simulink model "proto5"  (R2013b)
settings: Solver=ode45  StartTime=0.0  StopTime=3950  RelTol=1e-3
libraries: xbsIndex_r4 x1250, casper_library_misc x10, xps_library x3
(part 2 of 10)

== system proto5/1st_time ==
  out_reg : Inport
  assert_reg : xbsIndex_r4/Assert  assert_type=on  type_source=Explicitly  gui_display_data_type=Fixed-point  arith_type=Unsigned  n_bits=32  bin_pt=0  preci_type=Single  exp_width=8  frac_width=24  assert_rate=off  rate_source=Explicitly  period=1  output_port=on  block_type=assert
  cast_gw : xbsIndex_r4/Convert  gui_display_data_type=Fixed-point  arith_type=Unsigned  n_bits=32  bin_pt=0  float_type=Single  exp_bits=8  fraction_bits=24  quantization=Truncate  overflow=Wrap  en=off  latency=0  dbl_ovrd=off  pipeline=off  block_type=convert
  io_delay : xbsIndex_r4/Delay  rst=off  infoeditControl=Selection of Reset will increase slice count due to use of real FFs and instead of SRLs  en=off  latency=0  dbl_ovrd=off  reg_retiming=on  block_type=delay
  proto5_1st_time_user_data_in : xbsIndex_r4/Gateway Out  inherit_from_input=off  hdl_port=on  timing_constraint=None  locs_specified=off  LOCs={}  UseAsDAC=off  DACChannel='1'  block_type=gatewayout
  reint1 : xbsIndex_r4/Reinterpret  force_arith_type=on  arith_type=Unsigned  force_bin_pt=on  bin_pt=0  block_type=reinterpret
  sim_out : Terminator
  wires:
  io_delay/1 -> cast_gw/1
  cast_gw/1 -> proto5_1st_time_user_data_in/1
  proto5_1st_time_user_data_in/1 -> sim_out/1
  out_reg/1 -> assert_reg/1
  assert_reg/1 -> reint1/1
  reint1/1 -> io_delay/1

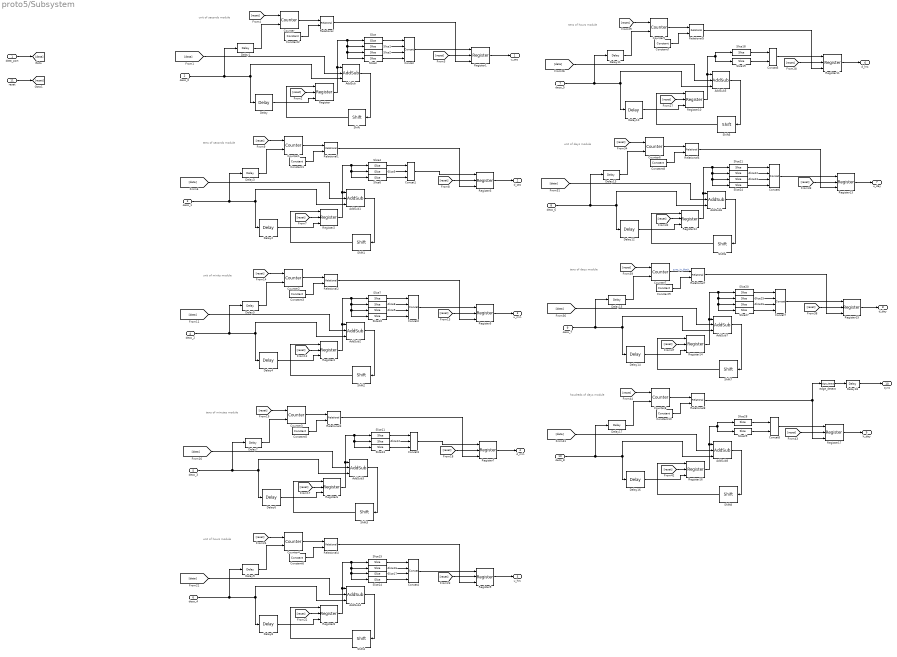
== system proto5/Subsystem ==
  note: unit of seconds module
  note: tens of seconds module
  note: unit of minits module
  note: tens of minutes module
  note: unit of hours module
  note: tens of hours module
  note: unit of days module
  note: tens of days module
  note: houdreds of days module
  data_port : Inport
  deco_0 : Inport  Port=2
  deco_1 : Inport  Port=3
  deco_2 : Inport  Port=4
  deco_3 : Inport  Port=5
  deco_4 : Inport  Port=6
  deco_5 : Inport  Port=7
  deco_6 : Inport  Port=8
  deco_7 : Inport  Port=9
  deco_8 : Inport  Port=10
  reset : Inport  Port=11
  AddSub{,2,4,6..7} (5 alike) : xbsIndex_r4/AddSub  mode=Addition  use_carryin=off  use_carryout=off  en=on  latency=1  precision=User Defined  arith_type=Unsigned  n_bits=5  bin_pt=0  quantization=Truncate  overflow=Wrap  dbl_ovrd=off  use_behavioral_HDL=off  hw_selection=Fabric  pipelined=off  block_type=addsub
  AddSub1 : xbsIndex_r4/AddSub  mode=Addition  use_carryin=off  use_carryout=off  en=on  latency=1  precision=User Defined  arith_type=Unsigned  n_bits=4  bin_pt=0  quantization=Truncate  overflow=Wrap  dbl_ovrd=off  use_behavioral_HDL=off  hw_selection=Fabric  pipelined=off  block_type=addsub
  AddSub3 : xbsIndex_r4/AddSub  mode=Addition  use_carryin=off  use_carryout=off  en=on  latency=1  precision=User Defined  arith_type=Unsigned  n_bits=4  bin_pt=0  quantization=Truncate  overflow=Wrap  dbl_ovrd=off  use_behavioral_HDL=off  hw_selection=Fabric  pipelined=off  block_type=addsub
  AddSub5 : xbsIndex_r4/AddSub  mode=Addition  use_carryin=off  use_carryout=off  en=on  latency=1  precision=User Defined  arith_type=Unsigned  n_bits=3  bin_pt=0  quantization=Truncate  overflow=Wrap  dbl_ovrd=off  use_behavioral_HDL=off  hw_selection=Fabric  pipelined=off  block_type=addsub
  AddSub8 : xbsIndex_r4/AddSub  mode=Addition  use_carryin=off  use_carryout=off  en=on  latency=1  precision=User Defined  arith_type=Unsigned  n_bits=3  bin_pt=0  quantization=Truncate  overflow=Wrap  dbl_ovrd=off  use_behavioral_HDL=off  hw_selection=Fabric  pipelined=off  block_type=addsub
  Concat{,2,4,6..7} (5 alike) : xbsIndex_r4/Concat  num_inputs=4  dbl_ovrd=off  block_type=concat
  Concat1 : xbsIndex_r4/Concat  num_inputs=3  dbl_ovrd=off  block_type=concat
  Concat3 : xbsIndex_r4/Concat  num_inputs=3  dbl_ovrd=off  block_type=concat
  Concat5 : xbsIndex_r4/Concat  num_inputs=2  dbl_ovrd=off  block_type=concat
  Concat8 : xbsIndex_r4/Concat  num_inputs=2  dbl_ovrd=off  block_type=concat
  Constant1 : xbsIndex_r4/Constant  const=3  gui_display_data_type=Fixed-point  arith_type=Unsigned  n_bits=4  bin_pt=0  preci_type=Single  exp_width=8  frac_width=24  explicit_period=on  period=1  equ=P=C  opselect=C  inp2=PCIN>>17  opr=+  inp1=P  carry=CIN  dbl_ovrd=off  block_type=constant
  Constant10 : xbsIndex_r4/Constant  const=2  gui_display_data_type=Fixed-point  arith_type=Unsigned  n_bits=3  bin_pt=0  preci_type=Single  exp_width=8  frac_width=24  explicit_period=on  period=1  equ=P=C  opselect=C  inp2=PCIN>>17  opr=+  inp1=P  carry=CIN  dbl_ovrd=off  block_type=constant
  Constant{2..3,6,8..9} (5 alike) : xbsIndex_r4/Constant  const=4  gui_display_data_type=Fixed-point  arith_type=Unsigned  n_bits=4  bin_pt=0  preci_type=Single  exp_width=8  frac_width=24  explicit_period=on  period=1  equ=P=C  opselect=C  inp2=PCIN>>17  opr=+  inp1=P  carry=CIN  dbl_ovrd=off  block_type=constant
  Constant5 : xbsIndex_r4/Constant  const=3  gui_display_data_type=Fixed-point  arith_type=Unsigned  n_bits=4  bin_pt=0  preci_type=Single  exp_width=8  frac_width=24  explicit_period=on  period=1  equ=P=C  opselect=C  inp2=PCIN>>17  opr=+  inp1=P  carry=CIN  dbl_ovrd=off  block_type=constant
  Constant7 : xbsIndex_r4/Constant  const=2  gui_display_data_type=Fixed-point  arith_type=Unsigned  n_bits=3  bin_pt=0  preci_type=Single  exp_width=8  frac_width=24  explicit_period=on  period=1  equ=P=C  opselect=C  inp2=PCIN>>17  opr=+  inp1=P  carry=CIN  dbl_ovrd=off  block_type=constant
  Counter{,1..8} (9 alike) : xbsIndex_r4/Counter  cnt_type=Free Running  cnt_to=Inf  operation=Up  start_count=0  cnt_by_val=1  arith_type=Unsigned  n_bits=4  bin_pt=0  load_pin=off  rst=on  en=on  explicit_period=on  period=1  dbl_ovrd=off  use_behavioral_HDL=off  implementation=Fabric  block_type=counter
  Delay{,1..18} (19 alike) : xbsIndex_r4/Delay  rst=off  infoeditControl=Selection of Reset will increase slice count due to use of real FFs and instead of SRLs  en=off  latency=1  dbl_ovrd=off  reg_retiming=off  block_type=delay
  Register{,1..17} (18 alike) : xbsIndex_r4/Register  init=0  rst=on  en=on  dbl_ovrd=off  block_type=register
  Relational{,1..8} (9 alike) : xbsIndex_r4/Relational  mode=a=b  en=off  latency=0  dbl_ovrd=off  block_type=relational
  Shift{,1..8} (9 alike) : xbsIndex_r4/Shift  shift_dir=Left  shift_bits=1  en=off  latency=0  precision=Full  arith_type="Signed  (2's comp)"  n_bits=16  bin_pt=14  quantization=Truncate  overflow=Wrap  dbl_ovrd=off  block_type=shift
  Slice{,4,7,11,15,18,20..21,28} (9 alike) : xbsIndex_r4/Slice  nbits=1  boolean_output=off  mode=Lower Bit Location + Width  bit1=0  base1=MSB of Input  bit0=1  base0=LSB of Input  dbl_ovrd=off  block_type=slice
  Slice{1,5,8,12,16,19,22,25,29} (9 alike) : xbsIndex_r4/Slice  nbits=1  boolean_output=off  mode=Lower Bit Location + Width  bit1=0  base1=MSB of Input  bit0=2  base0=LSB of Input  dbl_ovrd=off  block_type=slice
  Slice{3,10,14,24,27} (5 alike) : xbsIndex_r4/Slice  nbits=1  boolean_output=off  mode=Lower Bit Location + Width  bit1=0  base1=MSB of Input  bit0=4  base0=LSB of Input  dbl_ovrd=off  block_type=slice
  Slice{2,6,9,13,17,23,26} (7 alike) : xbsIndex_r4/Slice  nbits=1  boolean_output=off  mode=Lower Bit Location + Width  bit1=0  base1=MSB of Input  bit0=3  base0=LSB of Input  dbl_ovrd=off  block_type=slice
  edge_detect : casper_library_misc/edge_detect  edge=Rising  polarity=Active High  x_in=[0 0.08 0.08 0.16 0.16 0.24 0.24 0.32 0.32 0.4]  y_in="[-1 -1  1  1  1  1  1  1  1  1]"  x_out=[0.6 0.68 0.68 0.76 0.76 0.84 0.84 0.92 0.92 1]  y_out="[-1 -1  1  1 -1 -1 -1 -1 -1 -1]"
  u_sec : Outport
  d_sec : Outport  Port=2
  u_min : Outport  Port=3
  d_min : Outport  Port=4
  u_hrs : Outport  Port=5
  d_hrs : Outport  Port=6
  u_day : Outport  Port=7
  d_day : Outport  Port=8
  h_day : Outport  Port=9
  sync : Outport  Port=10
  wires:
  Constant7/1 -> Relational5/2
  Shift7/1 -> Register14/1
  Delay14/1 -> Register14/3
  [reset] -> Register10/2
  deco_5/1 -> Delay11/1, Delay10/1, AddSub5/3
  Register12/1 -> Slice24/1, Slice23/1, Slice22/1, Slice21/1, AddSub6/1
  Shift5/1 -> Register10/1
  Relational5/1 -> Register11/3
  [reset] -> Counter5/1
  Register15/1 -> d_day/1
  Delay15/1 -> Counter7/2
  [data] -> AddSub1/2
  Register13/1 -> u_day/1
  Delay13/1 -> Counter6/2
  Slice24/1 -> Concat6/4
  Register11/1 -> d_hrs/1
  [data] -> AddSub5/2
  AddSub5/1 -> Shift5/1
  Slice21/1 -> Concat6/1
  Slice23/1 -> Concat6/3
  Slice22/1 -> Concat6/2
  Register5/1 -> u_min/1
  Shift2/1 -> Register4/1
  [reset] -> Register3/2
  Slice7/1 -> Concat2/1
  Slice8/1 -> Concat2/2
  Delay6/1 -> Register6/3
  Slice12/1 -> Concat3/2
  [data] -> AddSub7/2
  [reset] -> Register11/2
  Register3/1 -> d_sec/1
  Counter7/1 -> Relational7/1  "sync_in_block"
  Delay/1 -> Register/3
  Slice/1 -> Concat/1
  Slice1/1 -> Concat/2
  Slice2/1 -> Concat/3
  Concat/1 -> Register1/1
  [reset] -> Counter/1
  Counter/1 -> Relational/1
  Constant2/1 -> Relational/2
  Relational/1 -> Register1/3
  [reset] -> Register1/2
  Register1/1 -> u_sec/1
  Delay1/1 -> Counter/2
  Slice6/1 -> Concat1/3
  [reset] -> Counter2/1
  Slice27/1 -> Concat7/4
  Slice20/1 -> Concat7/1
  Slice25/1 -> Concat7/2
  Slice26/1 -> Concat7/3
  Relational8/1 -> edge_detect/1, Register17/3
  [reset] -> Register17/2
  Register17/1 -> h_day/1
  Delay17/1 -> Counter8/2
  Register8/1 -> Slice14/1, Slice17/1, Slice16/1, Slice15/1, AddSub4/1
  [reset] -> Register12/2
  Shift6/1 -> Register12/1
  Delay12/1 -> Register12/3
  Delay10/1 -> Register10/3
  Slice29/1 -> Concat8/2
  Concat8/1 -> Register17/1
  [reset] -> Counter8/1
  Counter8/1 -> Relational8/1
  Constant10/1 -> Relational8/2
  AddSub8/1 -> Shift8/1
  Shift8/1 -> Register16/1
  Delay16/1 -> Register16/3
  Slice28/1 -> Concat8/1
  [reset] -> Register15/2
  deco_8/1 -> Delay17/1, AddSub8/3, Delay16/1
  [data] -> AddSub8/2
  [reset] -> Register16/2
  Register14/1 -> Slice27/1, Slice26/1, Slice25/1, Slice20/1, AddSub7/1
  Constant9/1 -> Relational7/2
  Relational7/1 -> Register15/3
  AddSub7/1 -> Shift7/1
  [reset] -> Register14/2
  Register16/1 -> Slice29/1, Slice28/1, AddSub8/1
  Register2/1 -> Slice6/1, Slice5/1, Slice4/1, AddSub1/1
  Constant5/1 -> Relational3/2
  [reset] -> Register7/2
  Slice19/1 -> Concat5/2
  [reset] -> Register2/2
  Constant1/1 -> Relational1/2
  AddSub2/1 -> Shift2/1
  [reset] -> Register4/2
  Concat7/1 -> Register15/1
  [reset] -> Counter7/1
  deco_2/1 -> Delay5/1, Delay4/1, AddSub2/3
  [data] -> AddSub3/2
  Delay4/1 -> Register4/3
  Slice9/1 -> Concat2/3
  Counter1/1 -> Relational1/1
  Counter5/1 -> Relational5/1
  Concat1/1 -> Register3/1
  Slice3/1 -> Concat/4
  Shift3/1 -> Register6/1
  AddSub3/1 -> Shift3/1
  Register10/1 -> Slice19/1, Slice18/1, AddSub5/1
  Relational2/1 -> Register5/3
  [reset] -> Register5/2
  AddSub1/1 -> Shift1/1
  Delay7/1 -> Counter3/2
  [data] -> AddSub6/2
  AddSub6/1 -> Shift6/1
  Relational3/1 -> Register7/3
  Register7/1 -> d_min/1
  deco_3/1 -> Delay7/1, Delay6/1, AddSub3/3
  Counter3/1 -> Relational3/1
  [reset] -> Counter3/1
  Slice10/1 -> Concat2/4
  Delay5/1 -> Counter2/2
  [data] -> AddSub2/2
  Relational1/1 -> Register3/3
  Counter2/1 -> Relational2/1
  Constant3/1 -> Relational2/2
  [reset] -> Register9/2
  Register9/1 -> u_hrs/1
  Delay9/1 -> Counter4/2
  Slice14/1 -> Concat4/4
  Register/1 -> Slice3/1, Slice2/1, Slice1/1, Slice/1, AddSub/1
  Register6/1 -> Slice13/1, Slice12/1, Slice11/1, AddSub3/1
  Concat2/1 -> Register5/1
  Delay3/1 -> Counter1/2
  Register4/1 -> Slice10/1, Slice9/1, Slice8/1, Slice7/1, AddSub2/1
  [reset] -> Counter4/1
  deco_6/1 -> Delay13/1, AddSub6/3, Delay12/1
  [data] -> AddSub4/2
  AddSub4/1 -> Shift4/1
  [reset] -> Register8/2
  deco_4/1 -> Delay9/1, Delay8/1, AddSub4/3
  Concat5/1 -> Register11/1
  Constant8/1 -> Relational6/2
  [reset] -> Register13/2
  Relational6/1 -> Register13/3
  Slice17/1 -> Concat4/3
  Constant6/1 -> Relational4/2
  Counter4/1 -> Relational4/1
  Relational4/1 -> Register9/3
  Delay11/1 -> Counter5/2
  Concat6/1 -> Register13/1
  Counter6/1 -> Relational6/1
  [reset] -> Counter6/1
  Slice18/1 -> Concat5/1
  deco_7/1 -> Delay15/1, Delay14/1, AddSub7/3
  Shift4/1 -> Register8/1
  Delay8/1 -> Register8/3
  Slice15/1 -> Concat4/1
  Concat4/1 -> Register9/1
  Slice16/1 -> Concat4/2
  Slice13/1 -> Concat3/3
  Concat3/1 -> Register7/1
  deco_1/1 -> Delay3/1, Delay2/1, AddSub1/3
  Delay2/1 -> Register2/3
  deco_0/1 -> Delay1/1, Delay/1, AddSub/3
  [data] -> AddSub/2
  AddSub/1 -> Shift/1
  [reset] -> Register/2
  Shift/1 -> Register/1
  Slice5/1 -> Concat1/2
  Shift1/1 -> Register2/1
  Slice4/1 -> Concat1/1
  [reset] -> Register6/2
  Slice11/1 -> Concat3/1
  [reset] -> Counter1/1
  data_port/1 -> [data]
  reset/1 -> [reset]
  edge_detect/1 -> Delay18/1
  Delay18/1 -> sync/1

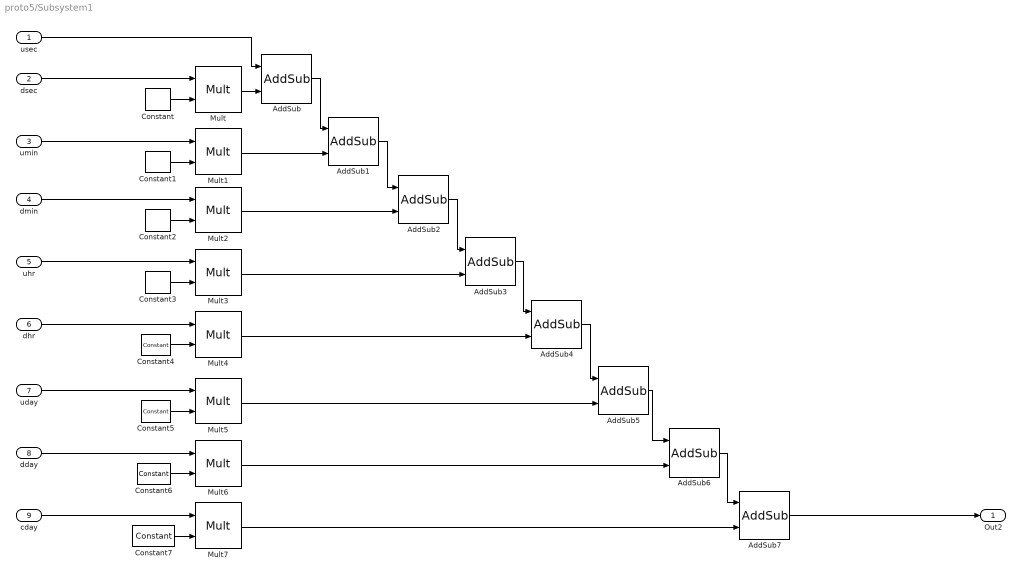
== system proto5/Subsystem1 ==
  usec : Inport
  dsec : Inport  Port=2
  umin : Inport  Port=3
  dmin : Inport  Port=4
  uhr : Inport  Port=5
  dhr : Inport  Port=6
  uday : Inport  Port=7
  dday : Inport  Port=8
  cday : Inport  Port=9
  AddSub{,1..7} (8 alike) : xbsIndex_r4/AddSub  mode=Addition  use_carryin=off  use_carryout=off  en=off  latency=2  precision=Full  arith_type=Unsigned  n_bits=16  bin_pt=14  quantization=Truncate  overflow=Wrap  dbl_ovrd=off  use_behavioral_HDL=off  hw_selection=DSP48  pipelined=off  block_type=addsub
  Constant : xbsIndex_r4/Constant  const=10  gui_display_data_type=Fixed-point  arith_type=Unsigned  n_bits=24  bin_pt=0  preci_type=Single  exp_width=8  frac_width=24  explicit_period=on  period=1  equ=P=C  opselect=C  inp2=PCIN>>17  opr=+  inp1=P  carry=CIN  dbl_ovrd=off  block_type=constant
  Constant1 : xbsIndex_r4/Constant  const=60  gui_display_data_type=Fixed-point  arith_type=Unsigned  n_bits=24  bin_pt=0  preci_type=Single  exp_width=8  frac_width=24  explicit_period=on  period=1  equ=P=C  opselect=C  inp2=PCIN>>17  opr=+  inp1=P  carry=CIN  dbl_ovrd=off  block_type=constant
  Constant2 : xbsIndex_r4/Constant  const=600  gui_display_data_type=Fixed-point  arith_type=Unsigned  n_bits=24  bin_pt=0  preci_type=Single  exp_width=8  frac_width=24  explicit_period=on  period=1  equ=P=C  opselect=C  inp2=PCIN>>17  opr=+  inp1=P  carry=CIN  dbl_ovrd=off  block_type=constant
  Constant3 : xbsIndex_r4/Constant  const=3600  gui_display_data_type=Fixed-point  arith_type=Unsigned  n_bits=24  bin_pt=0  preci_type=Single  exp_width=8  frac_width=24  explicit_period=on  period=1  equ=P=C  opselect=C  inp2=PCIN>>17  opr=+  inp1=P  carry=CIN  dbl_ovrd=off  block_type=constant
  Constant4 : xbsIndex_r4/Constant  const=36000  gui_display_data_type=Fixed-point  arith_type=Unsigned  n_bits=24  bin_pt=0  preci_type=Single  exp_width=8  frac_width=24  explicit_period=on  period=1  equ=P=C  opselect=C  inp2=PCIN>>17  opr=+  inp1=P  carry=CIN  dbl_ovrd=off  block_type=constant
  Constant5 : xbsIndex_r4/Constant  const=86400  gui_display_data_type=Fixed-point  arith_type=Unsigned  n_bits=24  bin_pt=0  preci_type=Single  exp_width=8  frac_width=24  explicit_period=on  period=1  equ=P=C  opselect=C  inp2=PCIN>>17  opr=+  inp1=P  carry=CIN  dbl_ovrd=off  block_type=constant
  Constant6 : xbsIndex_r4/Constant  const=864000  gui_display_data_type=Fixed-point  arith_type=Unsigned  n_bits=24  bin_pt=0  preci_type=Single  exp_width=8  frac_width=24  explicit_period=on  period=1  equ=P=C  opselect=C  inp2=PCIN>>17  opr=+  inp1=P  carry=CIN  dbl_ovrd=off  block_type=constant
  Constant7 : xbsIndex_r4/Constant  const=8640000  gui_display_data_type=Fixed-point  arith_type=Unsigned  n_bits=24  bin_pt=0  preci_type=Single  exp_width=8  frac_width=24  explicit_period=on  period=1  equ=P=C  opselect=C  inp2=PCIN>>17  opr=+  inp1=P  carry=CIN  dbl_ovrd=off  block_type=constant
  Mult{,1..7} (8 alike) : xbsIndex_r4/Mult  precision=Full  arith_type="Signed  (2's comp)"  n_bits=16  bin_pt=14  quantization=Truncate  overflow=Wrap  en=off  latency=3  dbl_ovrd=off  use_behavioral_HDL=off  opt=Speed  use_embedded=on  optimum_pipeline=off  pipeline=on  use_rpm=on  placement_style=Triangular  block_type=mult
  Out2 : Outport
  wires:
  dsec/1 -> Mult/1
  Constant/1 -> Mult/2
  umin/1 -> Mult1/1
  Constant1/1 -> Mult1/2
  dmin/1 -> Mult2/1
  Constant2/1 -> Mult2/2
  uhr/1 -> Mult3/1
  Constant3/1 -> Mult3/2
  dhr/1 -> Mult4/1
  Constant4/1 -> Mult4/2
  uday/1 -> Mult5/1
  Constant5/1 -> Mult5/2
  dday/1 -> Mult6/1
  Constant6/1 -> Mult6/2
  cday/1 -> Mult7/1
  Constant7/1 -> Mult7/2
  Mult/1 -> AddSub/2
  usec/1 -> AddSub/1
  Mult1/1 -> AddSub1/2
  AddSub/1 -> AddSub1/1
  Mult2/1 -> AddSub2/2
  AddSub1/1 -> AddSub2/1
  AddSub2/1 -> AddSub3/1
  Mult3/1 -> AddSub3/2
  AddSub3/1 -> AddSub4/1
  Mult4/1 -> AddSub4/2
  AddSub4/1 -> AddSub5/1
  Mult5/1 -> AddSub5/2
  AddSub5/1 -> AddSub6/1
  Mult6/1 -> AddSub6/2
  AddSub6/1 -> AddSub7/1
  Mult7/1 -> AddSub7/2
  AddSub7/1 -> Out2/1

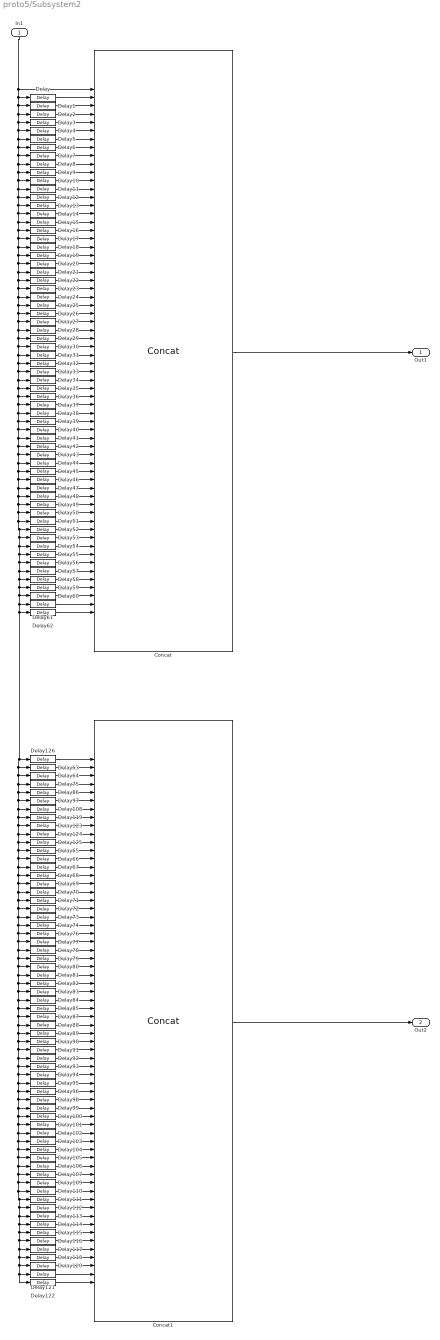
== system proto5/Subsystem2 ==
  In1 : Inport
  Concat : xbsIndex_r4/Concat  num_inputs=64  dbl_ovrd=off  block_type=concat
  Concat1 : xbsIndex_r4/Concat  num_inputs=64  dbl_ovrd=off  block_type=concat
  Delay : xbsIndex_r4/Delay  rst=off  infoeditControl=Selection of Reset will increase slice count due to use of real FFs and instead of SRLs  en=off  latency=1  dbl_ovrd=off  reg_retiming=off  block_type=delay
  Delay1 : xbsIndex_r4/Delay  rst=off  infoeditControl=Selection of Reset will increase slice count due to use of real FFs and instead of SRLs  en=off  latency=2  dbl_ovrd=off  reg_retiming=off  block_type=delay
  Delay10 : xbsIndex_r4/Delay  rst=off  infoeditControl=Selection of Reset will increase slice count due to use of real FFs and instead of SRLs  en=off  latency=11  dbl_ovrd=off  reg_retiming=off  block_type=delay
  Delay100 : xbsIndex_r4/Delay  rst=off  infoeditControl=Selection of Reset will increase slice count due to use of real FFs and instead of SRLs  en=off  latency=107  dbl_ovrd=off  reg_retiming=off  block_type=delay
  Delay101 : xbsIndex_r4/Delay  rst=off  infoeditControl=Selection of Reset will increase slice count due to use of real FFs and instead of SRLs  en=off  latency=108  dbl_ovrd=off  reg_retiming=off  block_type=delay
  Delay102 : xbsIndex_r4/Delay  rst=off  infoeditControl=Selection of Reset will increase slice count due to use of real FFs and instead of SRLs  en=off  latency=109  dbl_ovrd=off  reg_retiming=off  block_type=delay
  Delay103 : xbsIndex_r4/Delay  rst=off  infoeditControl=Selection of Reset will increase slice count due to use of real FFs and instead of SRLs  en=off  latency=110  dbl_ovrd=off  reg_retiming=off  block_type=delay
  Delay104 : xbsIndex_r4/Delay  rst=off  infoeditControl=Selection of Reset will increase slice count due to use of real FFs and instead of SRLs  en=off  latency=111  dbl_ovrd=off  reg_retiming=off  block_type=delay
  Delay105 : xbsIndex_r4/Delay  rst=off  infoeditControl=Selection of Reset will increase slice count due to use of real FFs and instead of SRLs  en=off  latency=112  dbl_ovrd=off  reg_retiming=off  block_type=delay
  Delay106 : xbsIndex_r4/Delay  rst=off  infoeditControl=Selection of Reset will increase slice count due to use of real FFs and instead of SRLs  en=off  latency=113  dbl_ovrd=off  reg_retiming=off  block_type=delay
  Delay107 : xbsIndex_r4/Delay  rst=off  infoeditControl=Selection of Reset will increase slice count due to use of real FFs and instead of SRLs  en=off  latency=114  dbl_ovrd=off  reg_retiming=off  block_type=delay
  Delay108 : xbsIndex_r4/Delay  rst=off  infoeditControl=Selection of Reset will increase slice count due to use of real FFs and instead of SRLs  en=off  latency=70  dbl_ovrd=off  reg_retiming=off  block_type=delay
  Delay109 : xbsIndex_r4/Delay  rst=off  infoeditControl=Selection of Reset will increase slice count due to use of real FFs and instead of SRLs  en=off  latency=115  dbl_ovrd=off  reg_retiming=off  block_type=delay
  Delay11 : xbsIndex_r4/Delay  rst=off  infoeditControl=Selection of Reset will increase slice count due to use of real FFs and instead of SRLs  en=off  latency=12  dbl_ovrd=off  reg_retiming=off  block_type=delay
  Delay110 : xbsIndex_r4/Delay  rst=off  infoeditControl=Selection of Reset will increase slice count due to use of real FFs and instead of SRLs  en=off  latency=116  dbl_ovrd=off  reg_retiming=off  block_type=delay
  Delay111 : xbsIndex_r4/Delay  rst=off  infoeditControl=Selection of Reset will increase slice count due to use of real FFs and instead of SRLs  en=off  latency=117  dbl_ovrd=off  reg_retiming=off  block_type=delay
  Delay112 : xbsIndex_r4/Delay  rst=off  infoeditControl=Selection of Reset will increase slice count due to use of real FFs and instead of SRLs  en=off  latency=118  dbl_ovrd=off  reg_retiming=off  block_type=delay
  Delay113 : xbsIndex_r4/Delay  rst=off  infoeditControl=Selection of Reset will increase slice count due to use of real FFs and instead of SRLs  en=off  latency=119  dbl_ovrd=off  reg_retiming=off  block_type=delay
  Delay114 : xbsIndex_r4/Delay  rst=off  infoeditControl=Selection of Reset will increase slice count due to use of real FFs and instead of SRLs  en=off  latency=120  dbl_ovrd=off  reg_retiming=off  block_type=delay
  Delay115 : xbsIndex_r4/Delay  rst=off  infoeditControl=Selection of Reset will increase slice count due to use of real FFs and instead of SRLs  en=off  latency=121  dbl_ovrd=off  reg_retiming=off  block_type=delay
  Delay116 : xbsIndex_r4/Delay  rst=off  infoeditControl=Selection of Reset will increase slice count due to use of real FFs and instead of SRLs  en=off  latency=122  dbl_ovrd=off  reg_retiming=off  block_type=delay
  Delay117 : xbsIndex_r4/Delay  rst=off  infoeditControl=Selection of Reset will increase slice count due to use of real FFs and instead of SRLs  en=off  latency=123  dbl_ovrd=off  reg_retiming=off  block_type=delay
  Delay118 : xbsIndex_r4/Delay  rst=off  infoeditControl=Selection of Reset will increase slice count due to use of real FFs and instead of SRLs  en=off  latency=124  dbl_ovrd=off  reg_retiming=off  block_type=delay
  Delay119 : xbsIndex_r4/Delay  rst=off  infoeditControl=Selection of Reset will increase slice count due to use of real FFs and instead of SRLs  en=off  latency=71  dbl_ovrd=off  reg_retiming=off  block_type=delay
  Delay12 : xbsIndex_r4/Delay  rst=off  infoeditControl=Selection of Reset will increase slice count due to use of real FFs and instead of SRLs  en=off  latency=13  dbl_ovrd=off  reg_retiming=off  block_type=delay
  Delay120 : xbsIndex_r4/Delay  rst=off  infoeditControl=Selection of Reset will increase slice count due to use of real FFs and instead of SRLs  en=off  latency=125  dbl_ovrd=off  reg_retiming=off  block_type=delay
  Delay121 : xbsIndex_r4/Delay  rst=off  infoeditControl=Selection of Reset will increase slice count due to use of real FFs and instead of SRLs  en=off  latency=126  dbl_ovrd=off  reg_retiming=off  block_type=delay
  Delay122 : xbsIndex_r4/Delay  rst=off  infoeditControl=Selection of Reset will increase slice count due to use of real FFs and instead of SRLs  en=off  latency=127  dbl_ovrd=off  reg_retiming=off  block_type=delay
  Delay123 : xbsIndex_r4/Delay  rst=off  infoeditControl=Selection of Reset will increase slice count due to use of real FFs and instead of SRLs  en=off  latency=72  dbl_ovrd=off  reg_retiming=off  block_type=delay
  Delay124 : xbsIndex_r4/Delay  rst=off  infoeditControl=Selection of Reset will increase slice count due to use of real FFs and instead of SRLs  en=off  latency=73  dbl_ovrd=off  reg_retiming=off  block_type=delay
  Delay125 : xbsIndex_r4/Delay  rst=off  infoeditControl=Selection of Reset will increase slice count due to use of real FFs and instead of SRLs  en=off  latency=74  dbl_ovrd=off  reg_retiming=off  block_type=delay
  Delay126 : xbsIndex_r4/Delay  rst=off  infoeditControl=Selection of Reset will increase slice count due to use of real FFs and instead of SRLs  en=off  latency=64  dbl_ovrd=off  reg_retiming=off  block_type=delay
  Delay13 : xbsIndex_r4/Delay  rst=off  infoeditControl=Selection of Reset will increase slice count due to use of real FFs and instead of SRLs  en=off  latency=14  dbl_ovrd=off  reg_retiming=off  block_type=delay
  Delay14 : xbsIndex_r4/Delay  rst=off  infoeditControl=Selection of Reset will increase slice count due to use of real FFs and instead of SRLs  en=off  latency=15  dbl_ovrd=off  reg_retiming=off  block_type=delay
  Delay15 : xbsIndex_r4/Delay  rst=off  infoeditControl=Selection of Reset will increase slice count due to use of real FFs and instead of SRLs  en=off  latency=16  dbl_ovrd=off  reg_retiming=off  block_type=delay
  Delay16 : xbsIndex_r4/Delay  rst=off  infoeditControl=Selection of Reset will increase slice count due to use of real FFs and instead of SRLs  en=off  latency=17  dbl_ovrd=off  reg_retiming=off  block_type=delay
  Delay17 : xbsIndex_r4/Delay  rst=off  infoeditControl=Selection of Reset will increase slice count due to use of real FFs and instead of SRLs  en=off  latency=18  dbl_ovrd=off  reg_retiming=off  block_type=delay
  Delay18 : xbsIndex_r4/Delay  rst=off  infoeditControl=Selection of Reset will increase slice count due to use of real FFs and instead of SRLs  en=off  latency=19  dbl_ovrd=off  reg_retiming=off  block_type=delay
  Delay19 : xbsIndex_r4/Delay  rst=off  infoeditControl=Selection of Reset will increase slice count due to use of real FFs and instead of SRLs  en=off  latency=20  dbl_ovrd=off  reg_retiming=off  block_type=delay
  Delay2 : xbsIndex_r4/Delay  rst=off  infoeditControl=Selection of Reset will increase slice count due to use of real FFs and instead of SRLs  en=off  latency=3  dbl_ovrd=off  reg_retiming=off  block_type=delay
  Delay20 : xbsIndex_r4/Delay  rst=off  infoeditControl=Selection of Reset will increase slice count due to use of real FFs and instead of SRLs  en=off  latency=21  dbl_ovrd=off  reg_retiming=off  block_type=delay
  Delay21 : xbsIndex_r4/Delay  rst=off  infoeditControl=Selection of Reset will increase slice count due to use of real FFs and instead of SRLs  en=off  latency=22  dbl_ovrd=off  reg_retiming=off  block_type=delay
  Delay22 : xbsIndex_r4/Delay  rst=off  infoeditControl=Selection of Reset will increase slice count due to use of real FFs and instead of SRLs  en=off  latency=23  dbl_ovrd=off  reg_retiming=off  block_type=delay
  Delay23 : xbsIndex_r4/Delay  rst=off  infoeditControl=Selection of Reset will increase slice count due to use of real FFs and instead of SRLs  en=off  latency=24  dbl_ovrd=off  reg_retiming=off  block_type=delay
  Delay24 : xbsIndex_r4/Delay  rst=off  infoeditControl=Selection of Reset will increase slice count due to use of real FFs and instead of SRLs  en=off  latency=25  dbl_ovrd=off  reg_retiming=off  block_type=delay
  Delay25 : xbsIndex_r4/Delay  rst=off  infoeditControl=Selection of Reset will increase slice count due to use of real FFs and instead of SRLs  en=off  latency=26  dbl_ovrd=off  reg_retiming=off  block_type=delay
  Delay26 : xbsIndex_r4/Delay  rst=off  infoeditControl=Selection of Reset will increase slice count due to use of real FFs and instead of SRLs  en=off  latency=27  dbl_ovrd=off  reg_retiming=off  block_type=delay
  Delay27 : xbsIndex_r4/Delay  rst=off  infoeditControl=Selection of Reset will increase slice count due to use of real FFs and instead of SRLs  en=off  latency=28  dbl_ovrd=off  reg_retiming=off  block_type=delay
  Delay28 : xbsIndex_r4/Delay  rst=off  infoeditControl=Selection of Reset will increase slice count due to use of real FFs and instead of SRLs  en=off  latency=29  dbl_ovrd=off  reg_retiming=off  block_type=delay
  Delay29 : xbsIndex_r4/Delay  rst=off  infoeditControl=Selection of Reset will increase slice count due to use of real FFs and instead of SRLs  en=off  latency=30  dbl_ovrd=off  reg_retiming=off  block_type=delay
  Delay3 : xbsIndex_r4/Delay  rst=off  infoeditControl=Selection of Reset will increase slice count due to use of real FFs and instead of SRLs  en=off  latency=4  dbl_ovrd=off  reg_retiming=off  block_type=delay
  Delay30 : xbsIndex_r4/Delay  rst=off  infoeditControl=Selection of Reset will increase slice count due to use of real FFs and instead of SRLs  en=off  latency=31  dbl_ovrd=off  reg_retiming=off  block_type=delay
  Delay31 : xbsIndex_r4/Delay  rst=off  infoeditControl=Selection of Reset will increase slice count due to use of real FFs and instead of SRLs  en=off  latency=32  dbl_ovrd=off  reg_retiming=off  block_type=delay
  Delay32 : xbsIndex_r4/Delay  rst=off  infoeditControl=Selection of Reset will increase slice count due to use of real FFs and instead of SRLs  en=off  latency=33  dbl_ovrd=off  reg_retiming=off  block_type=delay
  Delay33 : xbsIndex_r4/Delay  rst=off  infoeditControl=Selection of Reset will increase slice count due to use of real FFs and instead of SRLs  en=off  latency=34  dbl_ovrd=off  reg_retiming=off  block_type=delay
  Delay34 : xbsIndex_r4/Delay  rst=off  infoeditControl=Selection of Reset will increase slice count due to use of real FFs and instead of SRLs  en=off  latency=35  dbl_ovrd=off  reg_retiming=off  block_type=delay
  Delay35 : xbsIndex_r4/Delay  rst=off  infoeditControl=Selection of Reset will increase slice count due to use of real FFs and instead of SRLs  en=off  latency=36  dbl_ovrd=off  reg_retiming=off  block_type=delay
  Delay36 : xbsIndex_r4/Delay  rst=off  infoeditControl=Selection of Reset will increase slice count due to use of real FFs and instead of SRLs  en=off  latency=37  dbl_ovrd=off  reg_retiming=off  block_type=delay
  Delay37 : xbsIndex_r4/Delay  rst=off  infoeditControl=Selection of Reset will increase slice count due to use of real FFs and instead of SRLs  en=off  latency=38  dbl_ovrd=off  reg_retiming=off  block_type=delay
  Delay38 : xbsIndex_r4/Delay  rst=off  infoeditControl=Selection of Reset will increase slice count due to use of real FFs and instead of SRLs  en=off  latency=39  dbl_ovrd=off  reg_retiming=off  block_type=delay
  Delay39 : xbsIndex_r4/Delay  rst=off  infoeditControl=Selection of Reset will increase slice count due to use of real FFs and instead of SRLs  en=off  latency=40  dbl_ovrd=off  reg_retiming=off  block_type=delay
  Delay4 : xbsIndex_r4/Delay  rst=off  infoeditControl=Selection of Reset will increase slice count due to use of real FFs and instead of SRLs  en=off  latency=5  dbl_ovrd=off  reg_retiming=off  block_type=delay
  Delay40 : xbsIndex_r4/Delay  rst=off  infoeditControl=Selection of Reset will increase slice count due to use of real FFs and instead of SRLs  en=off  latency=41  dbl_ovrd=off  reg_retiming=off  block_type=delay
  Delay41 : xbsIndex_r4/Delay  rst=off  infoeditControl=Selection of Reset will increase slice count due to use of real FFs and instead of SRLs  en=off  latency=42  dbl_ovrd=off  reg_retiming=off  block_type=delay
  Delay42 : xbsIndex_r4/Delay  rst=off  infoeditControl=Selection of Reset will increase slice count due to use of real FFs and instead of SRLs  en=off  latency=43  dbl_ovrd=off  reg_retiming=off  block_type=delay
  Delay43 : xbsIndex_r4/Delay  rst=off  infoeditControl=Selection of Reset will increase slice count due to use of real FFs and instead of SRLs  en=off  latency=44  dbl_ovrd=off  reg_retiming=off  block_type=delay
  Delay44 : xbsIndex_r4/Delay  rst=off  infoeditControl=Selection of Reset will increase slice count due to use of real FFs and instead of SRLs  en=off  latency=45  dbl_ovrd=off  reg_retiming=off  block_type=delay
  Delay45 : xbsIndex_r4/Delay  rst=off  infoeditControl=Selection of Reset will increase slice count due to use of real FFs and instead of SRLs  en=off  latency=46  dbl_ovrd=off  reg_retiming=off  block_type=delay
  Delay46 : xbsIndex_r4/Delay  rst=off  infoeditControl=Selection of Reset will increase slice count due to use of real FFs and instead of SRLs  en=off  latency=47  dbl_ovrd=off  reg_retiming=off  block_type=delay
  Delay47 : xbsIndex_r4/Delay  rst=off  infoeditControl=Selection of Reset will increase slice count due to use of real FFs and instead of SRLs  en=off  latency=48  dbl_ovrd=off  reg_retiming=off  block_type=delay
  Delay48 : xbsIndex_r4/Delay  rst=off  infoeditControl=Selection of Reset will increase slice count due to use of real FFs and instead of SRLs  en=off  latency=49  dbl_ovrd=off  reg_retiming=off  block_type=delay
  Delay49 : xbsIndex_r4/Delay  rst=off  infoeditControl=Selection of Reset will increase slice count due to use of real FFs and instead of SRLs  en=off  latency=50  dbl_ovrd=off  reg_retiming=off  block_type=delay
  Delay5 : xbsIndex_r4/Delay  rst=off  infoeditControl=Selection of Reset will increase slice count due to use of real FFs and instead of SRLs  en=off  latency=6  dbl_ovrd=off  reg_retiming=off  block_type=delay
  Delay50 : xbsIndex_r4/Delay  rst=off  infoeditControl=Selection of Reset will increase slice count due to use of real FFs and instead of SRLs  en=off  latency=51  dbl_ovrd=off  reg_retiming=off  block_type=delay
  Delay51 : xbsIndex_r4/Delay  rst=off  infoeditControl=Selection of Reset will increase slice count due to use of real FFs and instead of SRLs  en=off  latency=52  dbl_ovrd=off  reg_retiming=off  block_type=delay
  Delay52 : xbsIndex_r4/Delay  rst=off  infoeditControl=Selection of Reset will increase slice count due to use of real FFs and instead of SRLs  en=off  latency=53  dbl_ovrd=off  reg_retiming=off  block_type=delay
  Delay53 : xbsIndex_r4/Delay  rst=off  infoeditControl=Selection of Reset will increase slice count due to use of real FFs and instead of SRLs  en=off  latency=54  dbl_ovrd=off  reg_retiming=off  block_type=delay
  Delay54 : xbsIndex_r4/Delay  rst=off  infoeditControl=Selection of Reset will increase slice count due to use of real FFs and instead of SRLs  en=off  latency=55  dbl_ovrd=off  reg_retiming=off  block_type=delay
  Delay55 : xbsIndex_r4/Delay  rst=off  infoeditControl=Selection of Reset will increase slice count due to use of real FFs and instead of SRLs  en=off  latency=56  dbl_ovrd=off  reg_retiming=off  block_type=delay
  Delay56 : xbsIndex_r4/Delay  rst=off  infoeditControl=Selection of Reset will increase slice count due to use of real FFs and instead of SRLs  en=off  latency=57  dbl_ovrd=off  reg_retiming=off  block_type=delay
  Delay57 : xbsIndex_r4/Delay  rst=off  infoeditControl=Selection of Reset will increase slice count due to use of real FFs and instead of SRLs  en=off  latency=58  dbl_ovrd=off  reg_retiming=off  block_type=delay
  Delay58 : xbsIndex_r4/Delay  rst=off  infoeditControl=Selection of Reset will increase slice count due to use of real FFs and instead of SRLs  en=off  latency=59  dbl_ovrd=off  reg_retiming=off  block_type=delay
  Delay59 : xbsIndex_r4/Delay  rst=off  infoeditControl=Selection of Reset will increase slice count due to use of real FFs and instead of SRLs  en=off  latency=60  dbl_ovrd=off  reg_retiming=off  block_type=delay
  Delay6 : xbsIndex_r4/Delay  rst=off  infoeditControl=Selection of Reset will increase slice count due to use of real FFs and instead of SRLs  en=off  latency=7  dbl_ovrd=off  reg_retiming=off  block_type=delay
  Delay60 : xbsIndex_r4/Delay  rst=off  infoeditControl=Selection of Reset will increase slice count due to use of real FFs and instead of SRLs  en=off  latency=61  dbl_ovrd=off  reg_retiming=off  block_type=delay
  Delay61 : xbsIndex_r4/Delay  rst=off  infoeditControl=Selection of Reset will increase slice count due to use of real FFs and instead of SRLs  en=off  latency=62  dbl_ovrd=off  reg_retiming=off  block_type=delay
  Delay62 : xbsIndex_r4/Delay  rst=off  infoeditControl=Selection of Reset will increase slice count due to use of real FFs and instead of SRLs  en=off  latency=63  dbl_ovrd=off  reg_retiming=off  block_type=delay
  Delay63 : xbsIndex_r4/Delay  rst=off  infoeditControl=Selection of Reset will increase slice count due to use of real FFs and instead of SRLs  en=off  latency=65  dbl_ovrd=off  reg_retiming=off  block_type=delay
  Delay64 : xbsIndex_r4/Delay  rst=off  infoeditControl=Selection of Reset will increase slice count due to use of real FFs and instead of SRLs  en=off  latency=66  dbl_ovrd=off  reg_retiming=off  block_type=delay
  Delay65 : xbsIndex_r4/Delay  rst=off  infoeditControl=Selection of Reset will increase slice count due to use of real FFs and instead of SRLs  en=off  latency=75  dbl_ovrd=off  reg_retiming=off  block_type=delay
  Delay66 : xbsIndex_r4/Delay  rst=off  infoeditControl=Selection of Reset will increase slice count due to use of real FFs and instead of SRLs  en=off  latency=76  dbl_ovrd=off  reg_retiming=off  block_type=delay
  Delay67 : xbsIndex_r4/Delay  rst=off  infoeditControl=Selection of Reset will increase slice count due to use of real FFs and instead of SRLs  en=off  latency=77  dbl_ovrd=off  reg_retiming=off  block_type=delay
  Delay68 : xbsIndex_r4/Delay  rst=off  infoeditControl=Selection of Reset will increase slice count due to use of real FFs and instead of SRLs  en=off  latency=78  dbl_ovrd=off  reg_retiming=off  block_type=delay
  Delay69 : xbsIndex_r4/Delay  rst=off  infoeditControl=Selection of Reset will increase slice count due to use of real FFs and instead of SRLs  en=off  latency=79  dbl_ovrd=off  reg_retiming=off  block_type=delay
  Delay7 : xbsIndex_r4/Delay  rst=off  infoeditControl=Selection of Reset will increase slice count due to use of real FFs and instead of SRLs  en=off  latency=8  dbl_ovrd=off  reg_retiming=off  block_type=delay
  Delay70 : xbsIndex_r4/Delay  rst=off  infoeditControl=Selection of Reset will increase slice count due to use of real FFs and instead of SRLs  en=off  latency=80  dbl_ovrd=off  reg_retiming=off  block_type=delay
  Delay71 : xbsIndex_r4/Delay  rst=off  infoeditControl=Selection of Reset will increase slice count due to use of real FFs and instead of SRLs  en=off  latency=81  dbl_ovrd=off  reg_retiming=off  block_type=delay
  Delay72 : xbsIndex_r4/Delay  rst=off  infoeditControl=Selection of Reset will increase slice count due to use of real FFs and instead of SRLs  en=off  latency=82  dbl_ovrd=off  reg_retiming=off  block_type=delay
  Delay73 : xbsIndex_r4/Delay  rst=off  infoeditControl=Selection of Reset will increase slice count due to use of real FFs and instead of SRLs  en=off  latency=83  dbl_ovrd=off  reg_retiming=off  block_type=delay
  Delay74 : xbsIndex_r4/Delay  rst=off  infoeditControl=Selection of Reset will increase slice count due to use of real FFs and instead of SRLs  en=off  latency=84  dbl_ovrd=off  reg_retiming=off  block_type=delay
  Delay75 : xbsIndex_r4/Delay  rst=off  infoeditControl=Selection of Reset will increase slice count due to use of real FFs and instead of SRLs  en=off  latency=67  dbl_ovrd=off  reg_retiming=off  block_type=delay
  Delay76 : xbsIndex_r4/Delay  rst=off  infoeditControl=Selection of Reset will increase slice count due to use of real FFs and instead of SRLs  en=off  latency=85  dbl_ovrd=off  reg_retiming=off  block_type=delay
  Delay77 : xbsIndex_r4/Delay  rst=off  infoeditControl=Selection of Reset will increase slice count due to use of real FFs and instead of SRLs  en=off  latency=86  dbl_ovrd=off  reg_retiming=off  block_type=delay
  Delay78 : xbsIndex_r4/Delay  rst=off  infoeditControl=Selection of Reset will increase slice count due to use of real FFs and instead of SRLs  en=off  latency=87  dbl_ovrd=off  reg_retiming=off  block_type=delay
  Delay79 : xbsIndex_r4/Delay  rst=off  infoeditControl=Selection of Reset will increase slice count due to use of real FFs and instead of SRLs  en=off  latency=88  dbl_ovrd=off  reg_retiming=off  block_type=delay
  Delay8 : xbsIndex_r4/Delay  rst=off  infoeditControl=Selection of Reset will increase slice count due to use of real FFs and instead of SRLs  en=off  latency=9  dbl_ovrd=off  reg_retiming=off  block_type=delay
  Delay80 : xbsIndex_r4/Delay  rst=off  infoeditControl=Selection of Reset will increase slice count due to use of real FFs and instead of SRLs  en=off  latency=89  dbl_ovrd=off  reg_retiming=off  block_type=delay
  Delay81 : xbsIndex_r4/Delay  rst=off  infoeditControl=Selection of Reset will increase slice count due to use of real FFs and instead of SRLs  en=off  latency=90  dbl_ovrd=off  reg_retiming=off  block_type=delay
  Delay82 : xbsIndex_r4/Delay  rst=off  infoeditControl=Selection of Reset will increase slice count due to use of real FFs and instead of SRLs  en=off  latency=91  dbl_ovrd=off  reg_retiming=off  block_type=delay
  Delay83 : xbsIndex_r4/Delay  rst=off  infoeditControl=Selection of Reset will increase slice count due to use of real FFs and instead of SRLs  en=off  latency=92  dbl_ovrd=off  reg_retiming=off  block_type=delay
  Delay84 : xbsIndex_r4/Delay  rst=off  infoeditControl=Selection of Reset will increase slice count due to use of real FFs and instead of SRLs  en=off  latency=93  dbl_ovrd=off  reg_retiming=off  block_type=delay
  Delay85 : xbsIndex_r4/Delay  rst=off  infoeditControl=Selection of Reset will increase slice count due to use of real FFs and instead of SRLs  en=off  latency=94  dbl_ovrd=off  reg_retiming=off  block_type=delay
  Delay86 : xbsIndex_r4/Delay  rst=off  infoeditControl=Selection of Reset will increase slice count due to use of real FFs and instead of SRLs  en=off  latency=68  dbl_ovrd=off  reg_retiming=off  block_type=delay
  Delay87 : xbsIndex_r4/Delay  rst=off  infoeditControl=Selection of Reset will increase slice count due to use of real FFs and instead of SRLs  en=off  latency=95  dbl_ovrd=off  reg_retiming=off  block_type=delay
  Delay88 : xbsIndex_r4/Delay  rst=off  infoeditControl=Selection of Reset will increase slice count due to use of real FFs and instead of SRLs  en=off  latency=96  dbl_ovrd=off  reg_retiming=off  block_type=delay
  Delay89 : xbsIndex_r4/Delay  rst=off  infoeditControl=Selection of Reset will increase slice count due to use of real FFs and instead of SRLs  en=off  latency=97  dbl_ovrd=off  reg_retiming=off  block_type=delay
  Delay9 : xbsIndex_r4/Delay  rst=off  infoeditControl=Selection of Reset will increase slice count due to use of real FFs and instead of SRLs  en=off  latency=10  dbl_ovrd=off  reg_retiming=off  block_type=delay
  Delay90 : xbsIndex_r4/Delay  rst=off  infoeditControl=Selection of Reset will increase slice count due to use of real FFs and instead of SRLs  en=off  latency=98  dbl_ovrd=off  reg_retiming=off  block_type=delay
  Delay91 : xbsIndex_r4/Delay  rst=off  infoeditControl=Selection of Reset will increase slice count due to use of real FFs and instead of SRLs  en=off  latency=99  dbl_ovrd=off  reg_retiming=off  block_type=delay
  Delay92 : xbsIndex_r4/Delay  rst=off  infoeditControl=Selection of Reset will increase slice count due to use of real FFs and instead of SRLs  en=off  latency=100  dbl_ovrd=off  reg_retiming=off  block_type=delay
  Delay93 : xbsIndex_r4/Delay  rst=off  infoeditControl=Selection of Reset will increase slice count due to use of real FFs and instead of SRLs  en=off  latency=101  dbl_ovrd=off  reg_retiming=off  block_type=delay
  Delay94 : xbsIndex_r4/Delay  rst=off  infoeditControl=Selection of Reset will increase slice count due to use of real FFs and instead of SRLs  en=off  latency=102  dbl_ovrd=off  reg_retiming=off  block_type=delay
  Delay95 : xbsIndex_r4/Delay  rst=off  infoeditControl=Selection of Reset will increase slice count due to use of real FFs and instead of SRLs  en=off  latency=103  dbl_ovrd=off  reg_retiming=off  block_type=delay
  Delay96 : xbsIndex_r4/Delay  rst=off  infoeditControl=Selection of Reset will increase slice count due to use of real FFs and instead of SRLs  en=off  latency=104  dbl_ovrd=off  reg_retiming=off  block_type=delay
  Delay97 : xbsIndex_r4/Delay  rst=off  infoeditControl=Selection of Reset will increase slice count due to use of real FFs and instead of SRLs  en=off  latency=69  dbl_ovrd=off  reg_retiming=off  block_type=delay
  Delay98 : xbsIndex_r4/Delay  rst=off  infoeditControl=Selection of Reset will increase slice count due to use of real FFs and instead of SRLs  en=off  latency=105  dbl_ovrd=off  reg_retiming=off  block_type=delay
  Delay99 : xbsIndex_r4/Delay  rst=off  infoeditControl=Selection of Reset will increase slice count due to use of real FFs and instead of SRLs  en=off  latency=106  dbl_ovrd=off  reg_retiming=off  block_type=delay
  Out1 : Outport
  Out2 : Outport  Port=2
  wires:
  Delay/1 -> Concat/2
  Delay1/1 -> Concat/3
  Delay2/1 -> Concat/4
  Delay3/1 -> Concat/5
  Delay4/1 -> Concat/6
  Delay5/1 -> Concat/7
  Delay6/1 -> Concat/8
  Delay7/1 -> Concat/9
  Delay8/1 -> Concat/10
  Delay9/1 -> Concat/11
  Delay10/1 -> Concat/12
  Delay11/1 -> Concat/13
  Delay12/1 -> Concat/14
  Delay13/1 -> Concat/15
  Delay14/1 -> Concat/16
  Delay15/1 -> Concat/17
  Delay16/1 -> Concat/18
  Delay17/1 -> Concat/19
  Delay18/1 -> Concat/20
  Delay19/1 -> Concat/21
  Delay20/1 -> Concat/22
  Delay21/1 -> Concat/23
  Delay22/1 -> Concat/24
  Delay23/1 -> Concat/25
  Delay24/1 -> Concat/26
  Delay25/1 -> Concat/27
  Delay26/1 -> Concat/28
  Delay27/1 -> Concat/29
  Delay28/1 -> Concat/30
  Delay29/1 -> Concat/31
  Delay30/1 -> Concat/32
  Delay31/1 -> Concat/33
  Delay32/1 -> Concat/34
  Delay33/1 -> Concat/35
  Delay34/1 -> Concat/36
  Delay35/1 -> Concat/37
  Delay36/1 -> Concat/38
  Delay37/1 -> Concat/39
  Delay38/1 -> Concat/40
  Delay39/1 -> Concat/41
  Delay40/1 -> Concat/42
  Delay41/1 -> Concat/43
  Delay42/1 -> Concat/44
  Delay43/1 -> Concat/45
  Delay44/1 -> Concat/46
  Delay45/1 -> Concat/47
  Delay46/1 -> Concat/48
  Delay47/1 -> Concat/49
  Delay48/1 -> Concat/50
  Delay49/1 -> Concat/51
  Delay50/1 -> Concat/52
  Delay51/1 -> Concat/53
  Delay52/1 -> Concat/54
  Delay53/1 -> Concat/55
  Delay54/1 -> Concat/56
  Delay55/1 -> Concat/57
  Delay56/1 -> Concat/58
  Delay57/1 -> Concat/59
  Delay58/1 -> Concat/60
  Delay59/1 -> Concat/61
  Delay60/1 -> Concat/62
  Delay61/1 -> Concat/63
  Delay62/1 -> Concat/64
  Concat/1 -> Out1/1
  In1/1 -> Concat/1, Delay47/1, Delay51/1, Delay52/1, Delay53/1, Delay55/1, Delay58/1, Delay59/1, Delay61/1, Delay126/1, Delay105/1, Delay110/1, Delay111/1, Delay112/1, Delay114/1, Delay117/1, Delay118/1, Delay122/1, Delay121/1, Delay120/1, Delay116/1, Delay115/1, Delay113/1, Delay109/1, Delay107/1, Delay106/1, Delay104/1, Delay103/1, Delay102/1, Delay101/1, Delay100/1, Delay99/1, Delay98/1, Delay96/1, Delay95/1, Delay94/1, Delay93/1, Delay92/1, Delay91/1, Delay90/1, Delay89/1, Delay88/1, Delay87/1, Delay85/1, Delay84/1, Delay83/1, Delay82/1, Delay81/1, Delay80/1, Delay79/1, Delay78/1, Delay77/1, Delay76/1, Delay74/1, Delay73/1, Delay72/1, Delay71/1, Delay70/1, Delay69/1, Delay68/1, Delay67/1, Delay66/1, Delay65/1, Delay125/1, Delay124/1, Delay123/1, Delay119/1, Delay108/1, Delay97/1, Delay86/1, Delay75/1, Delay64/1, Delay63/1, Delay62/1, Delay60/1, Delay57/1, Delay56/1, Delay54/1, Delay50/1, Delay49/1, Delay48/1, Delay46/1, Delay45/1, Delay44/1, Delay43/1, Delay42/1, Delay41/1, Delay40/1, Delay39/1, Delay38/1, Delay37/1, Delay36/1, Delay35/1, Delay34/1, Delay33/1, Delay32/1, Delay31/1, Delay30/1, Delay29/1, Delay28/1, Delay27/1, Delay26/1, Delay25/1, Delay24/1, Delay23/1, Delay22/1, Delay21/1, Delay20/1, Delay19/1, Delay18/1, Delay17/1, Delay16/1, Delay15/1, Delay14/1, Delay13/1, Delay12/1, Delay11/1, Delay10/1, Delay9/1, Delay8/1, Delay7/1, Delay6/1, Delay5/1, Delay4/1, Delay3/1, Delay2/1, Delay1/1, Delay/1
  Delay63/1 -> Concat1/2
  Delay64/1 -> Concat1/3
  Delay75/1 -> Concat1/4
  Delay86/1 -> Concat1/5
  Delay97/1 -> Concat1/6
  Delay108/1 -> Concat1/7
  Delay119/1 -> Concat1/8
  Delay123/1 -> Concat1/9
  Delay124/1 -> Concat1/10
  Delay125/1 -> Concat1/11
  Delay65/1 -> Concat1/12
  Delay66/1 -> Concat1/13
  Delay67/1 -> Concat1/14
  Delay68/1 -> Concat1/15
  Delay69/1 -> Concat1/16
  Delay70/1 -> Concat1/17
  Delay71/1 -> Concat1/18
  Delay72/1 -> Concat1/19
  Delay73/1 -> Concat1/20
  Delay74/1 -> Concat1/21
  Delay76/1 -> Concat1/22
  Delay77/1 -> Concat1/23
  Delay78/1 -> Concat1/24
  Delay79/1 -> Concat1/25
  Delay80/1 -> Concat1/26
  Delay81/1 -> Concat1/27
  Delay82/1 -> Concat1/28
  Delay83/1 -> Concat1/29
  Delay84/1 -> Concat1/30
  Delay85/1 -> Concat1/31
  Delay87/1 -> Concat1/32
  Delay88/1 -> Concat1/33
  Delay89/1 -> Concat1/34
  Delay90/1 -> Concat1/35
  Delay91/1 -> Concat1/36
  Delay92/1 -> Concat1/37
  Delay93/1 -> Concat1/38
  Delay94/1 -> Concat1/39
  Delay95/1 -> Concat1/40
  Delay96/1 -> Concat1/41
  Delay98/1 -> Concat1/42
  Delay99/1 -> Concat1/43
  Delay100/1 -> Concat1/44
  Delay101/1 -> Concat1/45
  Delay102/1 -> Concat1/46
  Delay103/1 -> Concat1/47
  Delay104/1 -> Concat1/48
  Delay105/1 -> Concat1/49
  Delay106/1 -> Concat1/50
  Delay107/1 -> Concat1/51
  Delay109/1 -> Concat1/52
  Delay110/1 -> Concat1/53
  Delay111/1 -> Concat1/54
  Delay112/1 -> Concat1/55
  Delay113/1 -> Concat1/56
  Delay114/1 -> Concat1/57
  Delay115/1 -> Concat1/58
  Delay116/1 -> Concat1/59
  Delay117/1 -> Concat1/60
  Delay118/1 -> Concat1/61
  Delay120/1 -> Concat1/62
  Delay121/1 -> Concat1/63
  Delay122/1 -> Concat1/64
  Concat1/1 -> Out2/1
  Delay126/1 -> Concat1/1
